simulink model "model_2D_Trefoil"  (R2022b)
settings: Solver=FixedStepAuto  StartTime=0.0  StopTime=15  FixedStep=0.01  RelTol=1e-3
settings Model: Creator=70952  LastModifiedBy=70952
settings SolverCC: AlgebraicLoopSolver=TrustRegion
settings DebuggingCC: UnconnectedInputMsg=warning  UnconnectedOutputMsg=warning  UnconnectedLineMsg=warning  SFMachineParentedDataDiag=warning
settings ModelReferenceCC: EnableRefExpFcnMdlSchedulingChecks=on
settings RTWCC: DLArmComputeVersion=19.05

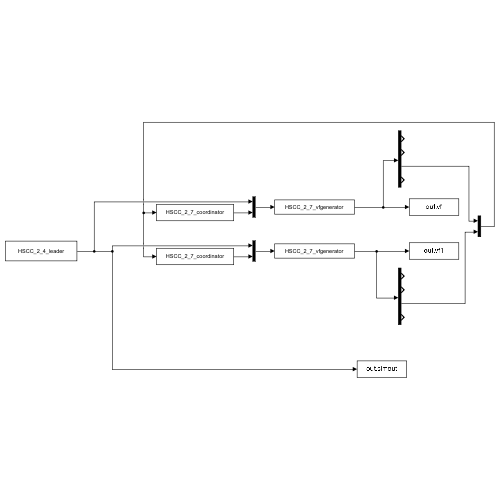
[thumbnail: Simulink's stored preview of the top-level diagram]
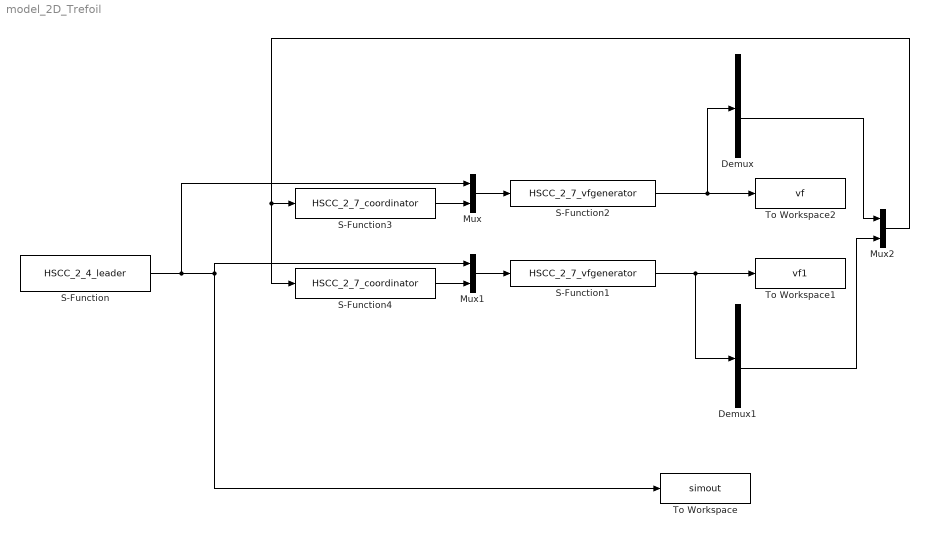
== system model_2D_Trefoil ==
  Demux : Demux
  Demux1 : Demux
  Mux : Mux  Inputs=2
  Mux1 : Mux  Inputs=2
  Mux2 : Mux  Inputs=2
  S-Function : S-Function  FunctionName=HSCC_2_4_leader  SFunctionDeploymentMode=off  EnableBusSupport=off
  S-Function1 : S-Function  FunctionName=HSCC_2_7_vfgenerator  Parameters=[1;-2;0]  SFunctionDeploymentMode=off  EnableBusSupport=off
  S-Function2 : S-Function  FunctionName=HSCC_2_7_vfgenerator  Parameters=[2;1;0]  SFunctionDeploymentMode=off  EnableBusSupport=off
  S-Function3 : S-Function  FunctionName=HSCC_2_7_coordinator  Parameters=[0 1;1 0],[0;0],1  SFunctionDeploymentMode=off  EnableBusSupport=off
  S-Function4 : S-Function  FunctionName=HSCC_2_7_coordinator  Parameters=[0 1;1 0],[0;0],2  SFunctionDeploymentMode=off  EnableBusSupport=off
  To Workspace : ToWorkspace  VariableName=simout  SampleTime=-1
  To Workspace1 : ToWorkspace  VariableName=vf1  SampleTime=-1
  To Workspace2 : ToWorkspace  VariableName=vf  SampleTime=-1
  wires:
  S-Function1/1 -> Demux1/1, To Workspace1/1
  S-Function/1 -> Mux/1, Mux1/1, To Workspace/1
  S-Function2/1 -> Demux/1, To Workspace2/1
  S-Function3/1 -> Mux/2
  Mux/1 -> S-Function2/1
  Mux1/1 -> S-Function1/1
  S-Function4/1 -> Mux1/2
  Demux1/3 -> Mux2/2
  Demux/3 -> Mux2/1
  Mux2/1 -> S-Function4/1, S-Function3/1
